simulink library "UXFD_Lib"  (R2016b)
settings: Solver=ode45  StartTime=0.0  StopTime=10.0  RelTol=1e-3  EnableMultiTasking=on
undefined symbols (not defined in the file): BreakpointData, BreakpointData1, BreakpointData2, BreakpointData_One_A, BreakpointData_Two_A, E2E_P01DataIDMode, E2E_P01ReceiverStatusType, EnumClass, iBit, initalValue, No_Runnable_Period, ObB_EidBsgStDerat_C, p_OVERRIDE_MASTER_SWITCH, SlDemoSign, SwitchOff_P, SwitchOn_P, Table, TableData_M, VCCTi33, VSysD_FidVehDerat1_C
libraries: simulink x28, CCMLib x11, UXFD_Lib x8, canmsglib x2, PTCC_Lib x1, hdlsllib x1
(part 5 of 7)

== system UXFD_Lib/Standard/Calibration/OverRide_with_master_switch ==
  override_value : Inport
  switch : Inport  Port=2
  input : Inport  Port=3
  Constant : Constant  Value=p_OVERRIDE_MASTER_SWITCH
  Constant1 : Constant  Value=85  OutDataTypeStr=uint8
  Data Type Conversion2 : DataTypeConversion  OutDataTypeStr=boolean
  Logical Operator : Logic
  Relational Operator1 : RelationalOperator  Operator===  OutDataTypeStr=boolean  RndMeth=Nearest  InputSameDT=on
  Switch1 : Switch  Criteria=u2 ~= 0  Threshold=1  RndMeth=Zero  InputSameDT=on
      settings: AttributesFormatString=%<Criteria>
  Out : Outport
  wires:
  Constant1/1 -> Relational Operator1/2
  Relational Operator1/1 -> Logical Operator/2
  input/1 -> Switch1/3
  Switch1/1 -> Out/1
  override_value/1 -> Switch1/1
  Data Type Conversion2/1 -> Switch1/2
  switch/1 -> Logical Operator/1
  Logical Operator/1 -> Data Type Conversion2/1
  Constant/1 -> Relational Operator1/1

== system UXFD_Lib/Standard/Calibration/xbackground1 ==

== system UXFD_Lib/Standard/Calibration/xbackground2 ==

== system UXFD_Lib/Standard/Calibration/xbackground3 ==

== system UXFD_Lib/Standard/Calibration/xbackground4 ==

== system UXFD_Lib/Standard/Discrete dynamics/BumplessRateTransfer ==
  s : Inport
  u1 : Inport  Port=2
  u0 : Inport  Port=3
  d10 : Inport  Port=4
  d01 : Inport  Port=5
  Add : Sum  Inputs=-+
  Add1 : Sum
  Constant1 : Constant  Value=0
  Constant2 : Constant
  LogicalSwitch1 : Subsystem  mask(GL_LogicSwitch_1.0){}
      mask init:
      | set_param(gcb,'LinkStatus','none');
      mask Display:
      | plot([-0.1 0.2 0.2], [0.85 0.85 0.75])
      | plot([-0.1 0.2 0.2], [0.5 0.5 0.6])
      | plot([0.8 1.1], [0.5 0.5])
      | plot([0.15 0.8], [0.6 0.5])
      | plot([-0.1 0.5 0.5], [0.15 0.15 0.6])
  Product : Product
  RateLimit : Subsystem  mask(PAG_Rate_Limiter_LV1.1_BV2){}
      mask help:
      | Rate limiter.
      | Limits the derivative of the input signal to a
      | value beween df (fall rate) and dr (rise rate).
      mask Display:
      | plot([0.35, 0.55, 0.55, 1.0], [0, 0, 1, 1])
      | plot([0.35, 0.55, 0.8, 1.0], [0, 0, 1, 1])
  Tq_EngInstReq_ : Outport
  wires:
  Add/1 -> Product/1
  Product/1 -> Add1/2
  Add1/1 -> Tq_EngInstReq_/1
  u0/1 -> Add1/1, Add/1
  u1/1 -> Add/2
  s/1 -> LogicalSwitch1/3(In3)
  Constant2/1 -> LogicalSwitch1/1(In1)
  Constant1/1 -> LogicalSwitch1/2(In2)
  d10/1 -> RateLimit/3(df)
  d01/1 -> RateLimit/2(dr)
  LogicalSwitch1/1(Out1) -> RateLimit/1(In1)
  RateLimit/1(y) -> Product/2

== system UXFD_Lib/Standard/Discrete dynamics/BumplessTransfer ==
  s : Inport
  u1 : Inport  Port=2
  u0 : Inport  Port=3
  tc : Inport  Port=4
  Add : Sum  Inputs=-+
  Add1 : Sum
  Constant : Constant  Value=0  OutDataTypeStr=Inherit: Inherit via back propagation
  Constant1 : Constant  OutDataTypeStr=Inherit: Inherit via back propagation
  LPF1_pole1 : Subsystem  mask(PAG_FirstOrder_Lowpass_Filter_LV1.1_BV2){}
      mask help:
      | Discrete low-pass filter. Corresponding analogue transfer function:
      |   1 / (1 + tau * s)
      mask Display:
      | plot([0.35, 0.9], [0, 0], [0.35, 0.35], [0, 1])
      | plot(0.35:0.55/10:0.9,   [0 0.39 0.63 0.78 0.86 0.92 0.95 0.98 0.99 0.99 0.99])
  LogicalSwitch1 : Subsystem  mask(GL_LogicSwitch_1.0){}
      mask init:
      | set_param(gcb,'LinkStatus','none');
      mask Display:
      | plot([-0.1 0.2 0.2], [0.85 0.85 0.75])
      | plot([-0.1 0.2 0.2], [0.5 0.5 0.6])
      | plot([0.8 1.1], [0.5 0.5])
      | plot([0.15 0.8], [0.6 0.5])
      | plot([-0.1 0.5 0.5], [0.15 0.15 0.6])
  Product : Product
  Out : Outport
  wires:
  Add/1 -> Product/1
  u0/1 -> Add1/1, Add/1
  s/1 -> LogicalSwitch1/3(In3)
  Product/1 -> Add1/2
  Add1/1 -> Out/1
  u1/1 -> Add/2
  LogicalSwitch1/1(Out1) -> LPF1_pole1/1(u)
  Constant1/1 -> LogicalSwitch1/1(In1)
  Constant/1 -> LogicalSwitch1/2(In2)
  LPF1_pole1/1(y) -> Product/2
  tc/1 -> LPF1_pole1/2(tc)

== system UXFD_Lib/Standard/Discrete dynamics/DLPF1_pole_v2 ==
  u : Inport
  tc : Inport  Port=2
  Add : Sum
  Add1 : Sum  Inputs=-+
  Add2 : Sum
  Add3 : Sum  Inputs=+-
  Constant : Constant  Value=0
  Constant1 : Constant  Value=0
  Constant2 : Constant  Value=1e-6
  Constant3 : Constant  Value=1e-6
  Divide : Product  Inputs=*/
  Divide1 : Product  Inputs=*/
  LogicalSwitch1 : Subsystem  mask(GL_LogicSwitch_1.0){}
      mask init:
      | set_param(gcb,'LinkStatus','none');
      mask Display:
      | plot([-0.1 0.2 0.2], [0.85 0.85 0.75])
      | plot([-0.1 0.2 0.2], [0.5 0.5 0.6])
      | plot([0.8 1.1], [0.5 0.5])
      | plot([0.15 0.8], [0.6 0.5])
      | plot([-0.1 0.5 0.5], [0.15 0.15 0.6])
  MinMax : MinMax  Function=max  Inputs=2
  MinMax1 : MinMax  Function=max  Inputs=2
  Product : Product
  Unit Delay : UnitDelay  SampleTime=-1
  Unit Delay1 : UnitDelay  SampleTime=-1
  Unit Delay2 : UnitDelay  SampleTime=-1
  ts : DataStoreRead  DataStoreName=ts
  y : Outport
  wires:
  tc/1 -> Add2/2
  MinMax1/1 -> Divide/2
  Constant3/1 -> MinMax1/2
  Add2/1 -> MinMax1/1
  u/1 -> Add3/1, Unit Delay/1
  Unit Delay/1 -> Add3/2
  Add3/1 -> Divide1/1
  Product/1 -> Add/2
  Divide1/1 -> Add1/2
  Unit Delay1/1 -> Add1/1, Add/1
  Divide/1 -> Product/2
  Add1/1 -> Product/1
  MinMax/1 -> Divide1/2
  Constant2/1 -> MinMax/2
  ts/1 -> Add2/1, MinMax/1, Divide/1
  Unit Delay2/1 -> LogicalSwitch1/3(In3)
  Constant1/1 -> Unit Delay2/1
  Constant/1 -> LogicalSwitch1/1(In1)
  Add/1 -> LogicalSwitch1/2(In2)
  LogicalSwitch1/1(Out1) -> Unit Delay1/1, y/1

== system UXFD_Lib/Standard/Discrete dynamics/FirstOrderFilter ==
  u : Inport
  tc : Inport  Port=2
  Constant1 : Constant  Value=1e-6  OutDataTypeStr=single  mask(TL_Constant){data={'output',{'type','Float32'},'date',735300.29228814819}}
      settings: CopyFcn=if exist('tl_reset_reviewflag','file')==2,tl_reset_reviewflag(gcbh);end  DeleteFcn=if exist('delete_tlblock','file')==2,delete_tlblock(gcbh);end  NameChangeFcn=if exist('rename_tlblock','file')==2,rename_tlblock(gcbh);end  OpenFcn=if exist('tl_open_blockdlg','file')==2,tl_open_blockdlg(gcbh);else,open_system(gcbh,'parameter');end
      mask Help: eval(['if exist(''tl_online_help'',''file'') == 2, tl_online_help(''Topic'',''TL_Constant''),else, web([''jar:file:///'',matlabroot,''/help/toolbox/simulink/help.jar!/slref/' lower(get_param(gcbh,'Blocktype')) '.html''], ''-helpbrowser''),end'])
      mask Display: plot([-0.05, 1.05, NaN, -0.05, 1.05],[.01, .01, NaN, .99, .99])
  Del1 : UnitDelay  SampleTime=-1  mask(TL_UnitDelay){data={'logdata',{'maxnumvals',4096,'plotchannels',[]},'output',{'type','Float32'},'state',{'type','Float32'},'date',735300.29228789348}}
      settings: CopyFcn=if exist('tl_reset_reviewflag','file')==2,tl_reset_reviewflag(gcbh);end  DeleteFcn=if exist('delete_tlblock','file')==2,delete_tlblock(gcbh);end  NameChangeFcn=if exist('rename_tlblock','file')==2,rename_tlblock(gcbh);end  OpenFcn=if exist('tl_open_blockdlg','file')==2,tl_open_blockdlg(gcbh);else,open_system(gcbh,'parameter');end
      mask Help: eval(['if exist(''tl_online_help'',''file'') == 2, tl_online_help(''Topic'',''TL_UnitDelay''),else, web([''jar:file:///'',matlabroot,''/help/toolbox/simulink/help.jar!/slref/' lower(get_param(gcbh,'Blocktype')) '.html''], ''-helpbrowser''),end'])
      mask Display: plot([-0.05, 1.05, NaN, -0.05, 1.05],[.01, .01, NaN, .99, .99])
  MinMax : MinMax  Function=max  Inputs=3  InputSameDT=on  mask(TL_MinMax){data={'logdata',{'maxnumvals',4096,'plotchannels',[]},'output',{'type','Float32'},'date',735300.29228754633}}
      settings: CopyFcn=if exist('tl_reset_reviewflag','file')==2,tl_reset_reviewflag(gcbh);end  DeleteFcn=if exist('delete_tlblock','file')==2,delete_tlblock(gcbh);end  NameChangeFcn=if exist('rename_tlblock','file')==2,rename_tlblock(gcbh);end  OpenFcn=if exist('tl_open_blockdlg','file')==2,tl_open_blockdlg(gcbh);else,open_system(gcbh,'parameter');end
      mask Help: eval(['if exist(''tl_online_help'',''file'') == 2, tl_online_help(''Topic'',''TL_MinMax''),else, web([''jar:file:///'',matlabroot,''/help/toolbox/simulink/help.jar!/slref/' lower(get_param(gcbh,'Blocktype')) '.html''], ''-helpbrowser''),end'])
      mask Display: plot([-0.05, 1.05, NaN, -0.05, 1.05],[.01, .01, NaN, .99, .99])
  Prod1 : Product  Inputs=*/  RndMeth=Zero  InputSameDT=on  OutDataTypeStr=Inherit: Same as first input  mask(TL_Product){data={'logdata',{'maxnumvals',4096,'plotchannels',[]},'output',{'type','Float32'},'date',735300.29228725692}}
      settings: CopyFcn=if exist('tl_reset_reviewflag','file')==2,tl_reset_reviewflag(gcbh);end  DeleteFcn=if exist('delete_tlblock','file')==2,delete_tlblock(gcbh);end  NameChangeFcn=if exist('rename_tlblock','file')==2,rename_tlblock(gcbh);end  OpenFcn=if exist('tl_open_blockdlg','file')==2,tl_open_blockdlg(gcbh);else,open_system(gcbh,'parameter');end
      mask Help: eval(['if exist(''tl_online_help'',''file'') == 2, tl_online_help(''Topic'',''TL_Product''),else, web([''jar:file:///'',matlabroot,''/help/toolbox/simulink/help.jar!/slref/' lower(get_param(gcbh,'Blocktype')) '.html''], ''-helpbrowser''),end'])
      mask Display: plot([-0.05, 1.05, NaN, -0.05, 1.05],[.01, .01, NaN, .99, .99])
  Prod2 : Product  RndMeth=Zero  InputSameDT=on  OutDataTypeStr=Inherit: Same as first input  mask(TL_Product){data={'logdata',{'maxnumvals',4096,'plotchannels',[]},'output',{'type','Float32'},'date',735300.29228697915}}
      settings: CopyFcn=if exist('tl_reset_reviewflag','file')==2,tl_reset_reviewflag(gcbh);end  DeleteFcn=if exist('delete_tlblock','file')==2,delete_tlblock(gcbh);end  NameChangeFcn=if exist('rename_tlblock','file')==2,rename_tlblock(gcbh);end  OpenFcn=if exist('tl_open_blockdlg','file')==2,tl_open_blockdlg(gcbh);else,open_system(gcbh,'parameter');end
      mask Help: eval(['if exist(''tl_online_help'',''file'') == 2, tl_online_help(''Topic'',''TL_Product''),else, web([''jar:file:///'',matlabroot,''/help/toolbox/simulink/help.jar!/slref/' lower(get_param(gcbh,'Blocktype')) '.html''], ''-helpbrowser''),end'])
      mask Display: plot([-0.05, 1.05, NaN, -0.05, 1.05],[.01, .01, NaN, .99, .99])
  Sum1 : Sum  Inputs=-+  InputSameDT=on  OutDataTypeStr=Inherit: Same as first input  mask(TL_Sum){data={'logdata',{'maxnumvals',4096,'plotchannels',[]},'output',{'type','Float32'},'date',735300.29228671291}}
      settings: CopyFcn=if exist('tl_reset_reviewflag','file')==2,tl_reset_reviewflag(gcbh);end  DeleteFcn=if exist('delete_tlblock','file')==2,delete_tlblock(gcbh);end  NameChangeFcn=if exist('rename_tlblock','file')==2,rename_tlblock(gcbh);end  OpenFcn=if exist('tl_open_blockdlg','file')==2,tl_open_blockdlg(gcbh);else,open_system(gcbh,'parameter');end
      mask Help: eval(['if exist(''tl_online_help'',''file'') == 2, tl_online_help(''Topic'',''TL_Sum''),else, web([''jar:file:///'',matlabroot,''/help/toolbox/simulink/help.jar!/slref/' lower(get_param(gcbh,'Blocktype')) '.html''], ''-helpbrowser''),end'])
      mask Display: plot([-0.05, 1.05, NaN, -0.05, 1.05],[.01, .01, NaN, .99, .99])
  Sum2 : Sum  InputSameDT=on  OutDataTypeStr=Inherit: Same as first input  mask(TL_Sum){data={'logdata',{'maxnumvals',4096,'plotchannels',[]},'output',{'type','Float32'},'date',735300.29228643514}}
      settings: CopyFcn=if exist('tl_reset_reviewflag','file')==2,tl_reset_reviewflag(gcbh);end  DeleteFcn=if exist('delete_tlblock','file')==2,delete_tlblock(gcbh);end  NameChangeFcn=if exist('rename_tlblock','file')==2,rename_tlblock(gcbh);end  OpenFcn=if exist('tl_open_blockdlg','file')==2,tl_open_blockdlg(gcbh);else,open_system(gcbh,'parameter');end
      mask Help: eval(['if exist(''tl_online_help'',''file'') == 2, tl_online_help(''Topic'',''TL_Sum''),else, web([''jar:file:///'',matlabroot,''/help/toolbox/simulink/help.jar!/slref/' lower(get_param(gcbh,'Blocktype')) '.html''], ''-helpbrowser''),end'])
      mask Display: plot([-0.05, 1.05, NaN, -0.05, 1.05],[.01, .01, NaN, .99, .99])
  ts : UXFD_Lib/Standard/Discrete dynamics/FirstOrderFilter1/ts  data={'logdata',{'plotchannels',[]},'date',735300.29228288191}
      settings: AttributesFormatString=ts
  y : Outport
  wires:
  u/1 -> Sum1/2
  Sum1/1 -> Prod2/1
  MinMax/1 -> Prod1/2
  ts/1 -> Prod1/1, MinMax/1
  Prod1/1 -> Prod2/2
  Del1/1 -> Sum1/1, Sum2/1
  Sum2/1 -> y/1, Del1/1
  tc/1 -> MinMax/2
  Prod2/1 -> Sum2/2
  Constant1/1 -> MinMax/3

== system UXFD_Lib/Standard/Discrete dynamics/FirstOrderFilter1 ==
  u : Inport
  r : Inport  Port=2
  rv : Inport  Port=3
  tc inc : Inport  Port=4
  tc dec : Inport  Port=5
  Constant : Constant  Value=0  mask(TL_Constant){data={'output',{'type','Float32'},'date',735300.29228606483}}
      settings: CopyFcn=if exist('tl_reset_reviewflag','file')==2,tl_reset_reviewflag(gcbh);end  DeleteFcn=if exist('delete_tlblock','file')==2,delete_tlblock(gcbh);end  NameChangeFcn=if exist('rename_tlblock','file')==2,rename_tlblock(gcbh);end  OpenFcn=if exist('tl_open_blockdlg','file')==2,tl_open_blockdlg(gcbh);else,open_system(gcbh,'parameter');end
      mask Help: eval(['if exist(''tl_online_help'',''file'') == 2, tl_online_help(''Topic'',''TL_Constant''),else, web([''jar:file:///'',matlabroot,''/help/toolbox/simulink/help.jar!/slref/' lower(get_param(gcbh,'Blocktype')) '.html''], ''-helpbrowser''),end'])
      mask Display: plot([-0.05, 1.05, NaN, -0.05, 1.05],[.01, .01, NaN, .99, .99])
  Constant1 : Constant  Value=1e-6  OutDataTypeStr=single  mask(TL_Constant){data={'output',{'type','Float32'},'date',735300.29228582175}}
      settings: CopyFcn=if exist('tl_reset_reviewflag','file')==2,tl_reset_reviewflag(gcbh);end  DeleteFcn=if exist('delete_tlblock','file')==2,delete_tlblock(gcbh);end  NameChangeFcn=if exist('rename_tlblock','file')==2,rename_tlblock(gcbh);end  OpenFcn=if exist('tl_open_blockdlg','file')==2,tl_open_blockdlg(gcbh);else,open_system(gcbh,'parameter');end
      mask Help: eval(['if exist(''tl_online_help'',''file'') == 2, tl_online_help(''Topic'',''TL_Constant''),else, web([''jar:file:///'',matlabroot,''/help/toolbox/simulink/help.jar!/slref/' lower(get_param(gcbh,'Blocktype')) '.html''], ''-helpbrowser''),end'])
      mask Display: plot([-0.05, 1.05, NaN, -0.05, 1.05],[.01, .01, NaN, .99, .99])
  Del1 : UnitDelay  SampleTime=-1  mask(TL_UnitDelay){data={'logdata',{'maxnumvals',4096,'plotchannels',[]},'output',{'type','Float32'},'state',{'type','Float32'},'date',735300.29228555551}}
      settings: CopyFcn=if exist('tl_reset_reviewflag','file')==2,tl_reset_reviewflag(gcbh);end  DeleteFcn=if exist('delete_tlblock','file')==2,delete_tlblock(gcbh);end  NameChangeFcn=if exist('rename_tlblock','file')==2,rename_tlblock(gcbh);end  OpenFcn=if exist('tl_open_blockdlg','file')==2,tl_open_blockdlg(gcbh);else,open_system(gcbh,'parameter');end
      mask Help: eval(['if exist(''tl_online_help'',''file'') == 2, tl_online_help(''Topic'',''TL_UnitDelay''),else, web([''jar:file:///'',matlabroot,''/help/toolbox/simulink/help.jar!/slref/' lower(get_param(gcbh,'Blocktype')) '.html''], ''-helpbrowser''),end'])
      mask Display: plot([-0.05, 1.05, NaN, -0.05, 1.05],[.01, .01, NaN, .99, .99])
  Demux : Demux  Outputs=2
  Max2 : MinMax  Function=max  Inputs=2  mask(TL_MinMax){data={'logdata',{'plotchannels',[]},'output',{'type','Float32'},'date',735300.29228521988}}
      settings: CopyFcn=if exist('tl_reset_reviewflag','file')==2,tl_reset_reviewflag(gcbh);end  DeleteFcn=if exist('delete_tlblock','file')==2,delete_tlblock(gcbh);end  NameChangeFcn=if exist('rename_tlblock','file')==2,rename_tlblock(gcbh);end  OpenFcn=if exist('tl_open_blockdlg','file')==2,tl_open_blockdlg(gcbh);else,open_system(gcbh,'parameter');end
      mask Help: eval(['if exist(''tl_online_help'',''file'') == 2, tl_online_help(''Topic'',''TL_MinMax''),else, web([''jar:file:///'',matlabroot,''/help/toolbox/simulink/help.jar!/slref/' lower(get_param(gcbh,'Blocktype')) '.html''], ''-helpbrowser''),end'])
      mask Display: plot([-0.05, 1.05, NaN, -0.05, 1.05],[.01, .01, NaN, .99, .99])
  Min : MinMax  Inputs=2  mask(TL_MinMax){data={'logdata',{'plotchannels',[]},'output',{'type','Float32'},'date',735300.29228494212}}
      settings: CopyFcn=if exist('tl_reset_reviewflag','file')==2,tl_reset_reviewflag(gcbh);end  DeleteFcn=if exist('delete_tlblock','file')==2,delete_tlblock(gcbh);end  NameChangeFcn=if exist('rename_tlblock','file')==2,rename_tlblock(gcbh);end  OpenFcn=if exist('tl_open_blockdlg','file')==2,tl_open_blockdlg(gcbh);else,open_system(gcbh,'parameter');end
      mask Help: eval(['if exist(''tl_online_help'',''file'') == 2, tl_online_help(''Topic'',''TL_MinMax''),else, web([''jar:file:///'',matlabroot,''/help/toolbox/simulink/help.jar!/slref/' lower(get_param(gcbh,'Blocktype')) '.html''], ''-helpbrowser''),end'])
      mask Display: plot([-0.05, 1.05, NaN, -0.05, 1.05],[.01, .01, NaN, .99, .99])
  MinMax : MinMax  Function=max  Inputs=3  InputSameDT=on  mask(TL_MinMax){data={'logdata',{'maxnumvals',4096,'plotchannels',[]},'output',{'type','Float32'},'date',735300.29228465282}}
      settings: CopyFcn=if exist('tl_reset_reviewflag','file')==2,tl_reset_reviewflag(gcbh);end  DeleteFcn=if exist('delete_tlblock','file')==2,delete_tlblock(gcbh);end  NameChangeFcn=if exist('rename_tlblock','file')==2,rename_tlblock(gcbh);end  OpenFcn=if exist('tl_open_blockdlg','file')==2,tl_open_blockdlg(gcbh);else,open_system(gcbh,'parameter');end
      mask Help: eval(['if exist(''tl_online_help'',''file'') == 2, tl_online_help(''Topic'',''TL_MinMax''),else, web([''jar:file:///'',matlabroot,''/help/toolbox/simulink/help.jar!/slref/' lower(get_param(gcbh,'Blocktype')) '.html''], ''-helpbrowser''),end'])
      mask Display: plot([-0.05, 1.05, NaN, -0.05, 1.05],[.01, .01, NaN, .99, .99])
  Mux : Mux  Inputs=2
  Mux1 : Mux  Inputs=2
  Prod1 : Product  Inputs=*/  RndMeth=Zero  InputSameDT=on  OutDataTypeStr=Inherit: Same as first input  mask(TL_Product){data={'logdata',{'maxnumvals',4096,'plotchannels',[]},'output',{'type','Float32'},'date',735300.29228437506}}
      settings: CopyFcn=if exist('tl_reset_reviewflag','file')==2,tl_reset_reviewflag(gcbh);end  DeleteFcn=if exist('delete_tlblock','file')==2,delete_tlblock(gcbh);end  NameChangeFcn=if exist('rename_tlblock','file')==2,rename_tlblock(gcbh);end  OpenFcn=if exist('tl_open_blockdlg','file')==2,tl_open_blockdlg(gcbh);else,open_system(gcbh,'parameter');end
      mask Help: eval(['if exist(''tl_online_help'',''file'') == 2, tl_online_help(''Topic'',''TL_Product''),else, web([''jar:file:///'',matlabroot,''/help/toolbox/simulink/help.jar!/slref/' lower(get_param(gcbh,'Blocktype')) '.html''], ''-helpbrowser''),end'])
      mask Display: plot([-0.05, 1.05, NaN, -0.05, 1.05],[.01, .01, NaN, .99, .99])
  Prod2 : Product  RndMeth=Zero  InputSameDT=on  OutDataTypeStr=Inherit: Same as first input  mask(TL_Product){data={'logdata',{'maxnumvals',4096,'plotchannels',[]},'output',{'type','Float32'},'date',735300.29228409717}}
      settings: CopyFcn=if exist('tl_reset_reviewflag','file')==2,tl_reset_reviewflag(gcbh);end  DeleteFcn=if exist('delete_tlblock','file')==2,delete_tlblock(gcbh);end  NameChangeFcn=if exist('rename_tlblock','file')==2,rename_tlblock(gcbh);end  OpenFcn=if exist('tl_open_blockdlg','file')==2,tl_open_blockdlg(gcbh);else,open_system(gcbh,'parameter');end
      mask Help: eval(['if exist(''tl_online_help'',''file'') == 2, tl_online_help(''Topic'',''TL_Product''),else, web([''jar:file:///'',matlabroot,''/help/toolbox/simulink/help.jar!/slref/' lower(get_param(gcbh,'Blocktype')) '.html''], ''-helpbrowser''),end'])
      mask Display: plot([-0.05, 1.05, NaN, -0.05, 1.05],[.01, .01, NaN, .99, .99])
  Sum1 : Sum  Inputs=-+  InputSameDT=on  OutDataTypeStr=Inherit: Same as first input  mask(TL_Sum){data={'logdata',{'maxnumvals',4096,'plotchannels',[]},'output',{'type','Float32'},'date',735300.29228373838}}
      settings: CopyFcn=if exist('tl_reset_reviewflag','file')==2,tl_reset_reviewflag(gcbh);end  DeleteFcn=if exist('delete_tlblock','file')==2,delete_tlblock(gcbh);end  NameChangeFcn=if exist('rename_tlblock','file')==2,rename_tlblock(gcbh);end  OpenFcn=if exist('tl_open_blockdlg','file')==2,tl_open_blockdlg(gcbh);else,open_system(gcbh,'parameter');end
      mask Help: eval(['if exist(''tl_online_help'',''file'') == 2, tl_online_help(''Topic'',''TL_Sum''),else, web([''jar:file:///'',matlabroot,''/help/toolbox/simulink/help.jar!/slref/' lower(get_param(gcbh,'Blocktype')) '.html''], ''-helpbrowser''),end'])
      mask Display: plot([-0.05, 1.05, NaN, -0.05, 1.05],[.01, .01, NaN, .99, .99])
  Sum2 : Sum  Inputs=+++  InputSameDT=on  OutDataTypeStr=Inherit: Same as first input  mask(TL_Sum){data={'logdata',{'maxnumvals',4096,'plotchannels',[]},'output',{'type','Float32'},'date',735300.29228347226}}
      settings: CopyFcn=if exist('tl_reset_reviewflag','file')==2,tl_reset_reviewflag(gcbh);end  DeleteFcn=if exist('delete_tlblock','file')==2,delete_tlblock(gcbh);end  NameChangeFcn=if exist('rename_tlblock','file')==2,rename_tlblock(gcbh);end  OpenFcn=if exist('tl_open_blockdlg','file')==2,tl_open_blockdlg(gcbh);else,open_system(gcbh,'parameter');end
      mask Help: eval(['if exist(''tl_online_help'',''file'') == 2, tl_online_help(''Topic'',''TL_Sum''),else, web([''jar:file:///'',matlabroot,''/help/toolbox/simulink/help.jar!/slref/' lower(get_param(gcbh,'Blocktype')) '.html''], ''-helpbrowser''),end'])
      mask Display: plot([-0.05, 1.05, NaN, -0.05, 1.05],[.01, .01, NaN, .99, .99])
  Switch : Switch  Criteria=u2 ~= 0  Threshold=0.5  mask(TL_Switch){data={'logdata',{'plotchannels',[]},'output',{'type','Float32'},'date',735300.29228318285}}
      settings: CopyFcn=if exist('tl_reset_reviewflag','file')==2,tl_reset_reviewflag(gcbh);end  DeleteFcn=if exist('delete_tlblock','file')==2,delete_tlblock(gcbh);end  NameChangeFcn=if exist('rename_tlblock','file')==2,rename_tlblock(gcbh);end  OpenFcn=if exist('tl_open_blockdlg','file')==2,tl_open_blockdlg(gcbh);else,open_system(gcbh,'parameter');end
      mask Help: eval(['if exist(''tl_online_help'',''file'') == 2, tl_online_help(''Topic'',''TL_Switch''),else, web([''jar:file:///'',matlabroot,''/help/toolbox/simulink/help.jar!/slref/' lower(get_param(gcbh,'Blocktype')) '.html''], ''-helpbrowser''),end'])
      mask Display: plot([-0.05, 1.05, NaN, -0.05, 1.05],[.01, .01, NaN, .99, .99])
  ts : DataStoreRead  DataStoreName=ts  mask(TL_DataStoreRead){data={'logdata',{'plotchannels',[]},'date',735300.29228288191}}
      settings: AttributesFormatString=ts  DeleteFcn=if exist('delete_tlblock','file')==2,delete_tlblock(gcbh);end  NameChangeFcn=if exist('rename_tlblock','file')==2,rename_tlblock(gcbh);end  OpenFcn=if exist('tl_open_blockdlg','file')==2,tl_open_blockdlg(gcbh);else,open_system(gcbh,'parameter');end
      mask Help: eval(['if exist(''tl_online_help'',''file'') == 2, tl_online_help(''Topic'',''TL_DataStoreRead''),else, web([''jar:file:///'',matlabroot,''/help/toolbox/simulink/help.jar!/slref/' lower(get_param(gcbh,'Blocktype')) '.html''], ''-helpbrowser''),end'])
      mask Display: plot([-0.05, 1.05, NaN, -0.05, 1.05],[.01, .01, NaN, .99, .99])
  y : Outport
  wires:
  Del1/1 -> Sum2/1, Sum1/1
  Prod1/1 -> Prod2/2
  ts/1 -> Prod1/1, MinMax/1
  MinMax/1 -> Prod1/2
  Sum1/1 -> Prod2/1
  u/1 -> Sum1/2
  tc inc/1 -> Mux/1
  tc dec/1 -> Mux/2
  Constant1/1 -> Mux1/1, Mux1/2
  Prod2/1 -> Demux/1
  Demux/1 -> Max2/1
  Demux/2 -> Min/2
  Constant/1 -> Max2/2, Min/1
  Max2/1 -> Sum2/2
  Min/1 -> Sum2/3
  Sum2/1 -> Switch/3
  rv/1 -> Switch/1
  r/1 -> Switch/2
  Switch/1 -> Del1/1, y/1
  Mux/1 -> MinMax/2
  Mux1/1 -> MinMax/3

== system UXFD_Lib/Standard/Discrete dynamics/HysteresisFilter ==
  note: Filter to avoid occilation during low slipp
      | when converter character is steep
  n_Eng5 : Inport
  n_Eng1 : Inport  Port=2
  Add : Sum
  Add1 : Sum  Inputs=+-
  Saturation1 : Subsystem  mask(GL_Saturation_1.0){}
      mask help:
      | If input_1 > input_2
      |   output = input_2
      | elseif input_1 < input_3
      |   output = input_3
      | else
      |   output = input_1
      |
      | Note that if the lower limit is set above the upper limit, the output will take the value of the input to the lower limit port.
      mask init:
      | set_param(gcb,'LinkStatus','none');
      mask Display: plot([0.3, 0.5, 0.7, 0.9], [0, 0, 1, 1])
  Unit Delay : UnitDelay  SampleTime=-1
  y : Outport
  wires:
  n_Eng5/1 -> Add/1, Add1/1
  Add1/1 -> Saturation1/3(L)
  Add/1 -> Saturation1/2(U)
  Saturation1/1(y) -> Unit Delay/1, y/1
  Unit Delay/1 -> Saturation1/1(u)
  n_Eng1/1 -> Add/2, Add1/2

== system UXFD_Lib/Standard/Discrete dynamics/LPF1_discreteReset ==
  u : Inport
  a : Inport  Port=2
  r : Inport  Port=3
  LogicalSwitch1 : Subsystem  mask(PAG_Switch_LV1.6_BV2){}
      mask help:
      | Pass through input 1 when input 3 is true;
      | otherwise, pass through input 2
      mask Display:
      | plot([-0.1 0.2 0.2], [0.85 0.85 0.75])
      | plot([-0.1 0.2 0.2], [0.5 0.5 0.6])
      | plot([0.8 1.1], [0.5 0.5])
      | plot([0.15 0.8], [0.6 0.5])
      | plot([-0.1 0.5 0.5], [0.15 0.15 0.6])
  Product : Product  SaturateOnIntegerOverflow=on  RndMeth=Zero  InputSameDT=on  OutDataTypeStr=Inherit: Same as first input  mask(TL_Product){data={'logdata',{'maxnumvals',4096,'plotchannels',[]},'output',{'type','Float32'},'date',735300.29228090274}}
      settings: CopyFcn=if exist('tl_reset_reviewflag','file')==2,tl_reset_reviewflag(gcbh);end  DeleteFcn=if exist('delete_tlblock','file')==2,delete_tlblock(gcbh);end  NameChangeFcn=if exist('rename_tlblock','file')==2,rename_tlblock(gcbh);end  OpenFcn=if exist('tl_open_blockdlg','file')==2,tl_open_blockdlg(gcbh);else,open_system(gcbh,'parameter');end
      mask Help: eval(['if exist(''tl_online_help'',''file'') == 2, tl_online_help(''Topic'',''TL_Product''),else, web([''jar:file:///'',matlabroot,''/help/toolbox/simulink/help.jar!/slref/' lower(get_param(gcbh,'Blocktype')) '.html''], ''-helpbrowser''),end'])
      mask Display: plot([-0.05, 1.05, NaN, -0.05, 1.05],[.01, .01, NaN, .99, .99])
  Sum : Sum  Inputs=+-  SaturateOnIntegerOverflow=on  InputSameDT=on  OutDataTypeStr=Inherit: Same as first input  mask(TL_Sum){data={'logdata',{'maxnumvals',4096,'plotchannels',[]},'output',{'type','Float32'},'date',735300.29228062497}}
      settings: CopyFcn=if exist('tl_reset_reviewflag','file')==2,tl_reset_reviewflag(gcbh);end  DeleteFcn=if exist('delete_tlblock','file')==2,delete_tlblock(gcbh);end  NameChangeFcn=if exist('rename_tlblock','file')==2,rename_tlblock(gcbh);end  OpenFcn=if exist('tl_open_blockdlg','file')==2,tl_open_blockdlg(gcbh);else,open_system(gcbh,'parameter');end
      mask Help: eval(['if exist(''tl_online_help'',''file'') == 2, tl_online_help(''Topic'',''TL_Sum''),else, web([''jar:file:///'',matlabroot,''/help/toolbox/simulink/help.jar!/slref/' lower(get_param(gcbh,'Blocktype')) '.html''], ''-helpbrowser''),end'])
      mask Display: plot([-0.05, 1.05, NaN, -0.05, 1.05],[.01, .01, NaN, .99, .99])
  Sum1 : Sum  SaturateOnIntegerOverflow=on  InputSameDT=on  OutDataTypeStr=Inherit: Same as first input  mask(TL_Sum){data={'logdata',{'maxnumvals',4096,'plotchannels',[]},'output',{'type','Float32'},'date',735300.2922803472}}
      settings: CopyFcn=if exist('tl_reset_reviewflag','file')==2,tl_reset_reviewflag(gcbh);end  DeleteFcn=if exist('delete_tlblock','file')==2,delete_tlblock(gcbh);end  NameChangeFcn=if exist('rename_tlblock','file')==2,rename_tlblock(gcbh);end  OpenFcn=if exist('tl_open_blockdlg','file')==2,tl_open_blockdlg(gcbh);else,open_system(gcbh,'parameter');end
      mask Help: eval(['if exist(''tl_online_help'',''file'') == 2, tl_online_help(''Topic'',''TL_Sum''),else, web([''jar:file:///'',matlabroot,''/help/toolbox/simulink/help.jar!/slref/' lower(get_param(gcbh,'Blocktype')) '.html''], ''-helpbrowser''),end'])
      mask Display: plot([-0.05, 1.05, NaN, -0.05, 1.05],[.01, .01, NaN, .99, .99])
  UnitDelay : UnitDelay  SampleTime=-1  mask(TL_UnitDelay){data={'logdata',{'maxnumvals',4096,'plotchannels',[]},'output',{'type','Float32'},'state',{'type','Float32'},'date',735300.29228006944}}
      settings: CopyFcn=if exist('tl_reset_reviewflag','file')==2,tl_reset_reviewflag(gcbh);end  DeleteFcn=if exist('delete_tlblock','file')==2,delete_tlblock(gcbh);end  NameChangeFcn=if exist('rename_tlblock','file')==2,rename_tlblock(gcbh);end  OpenFcn=if exist('tl_open_blockdlg','file')==2,tl_open_blockdlg(gcbh);else,open_system(gcbh,'parameter');end
      mask Help: eval(['if exist(''tl_online_help'',''file'') == 2, tl_online_help(''Topic'',''TL_UnitDelay''),else, web([''jar:file:///'',matlabroot,''/help/toolbox/simulink/help.jar!/slref/' lower(get_param(gcbh,'Blocktype')) '.html''], ''-helpbrowser''),end'])
      mask Display: plot([-0.05, 1.05, NaN, -0.05, 1.05],[.01, .01, NaN, .99, .99])
  y : Outport
  wires:
  Product/1 -> Sum1/1
  a/1 -> Product/2
  Sum/1 -> Product/1
  u/1 -> Sum/2, Sum1/2, LogicalSwitch1/1(In1)
  r/1 -> LogicalSwitch1/3(In2)
  UnitDelay/1 -> Sum/1
  Sum1/1 -> LogicalSwitch1/2(In3)
  LogicalSwitch1/1(Out1) -> y/1, UnitDelay/1

== system UXFD_Lib/Standard/Discrete dynamics/LPF2_discrete ==
  u : Inport
  a1 : Inport  Port=2
  a2 : Inport  Port=3
  b0 : Inport  Port=4
  b1 : Inport  Port=5
  b2 : Inport  Port=6
  Product : Product  SaturateOnIntegerOverflow=on  RndMeth=Zero  InputSameDT=on  OutDataTypeStr=Inherit: Same as first input  mask(TL_Product){data={'logdata',{'maxnumvals',4096,'plotchannels',[]},'output',{'type','Float32'},'date',735300.29227971064}}
      settings: CopyFcn=if exist('tl_reset_reviewflag','file')==2,tl_reset_reviewflag(gcbh);end  DeleteFcn=if exist('delete_tlblock','file')==2,delete_tlblock(gcbh);end  NameChangeFcn=if exist('rename_tlblock','file')==2,rename_tlblock(gcbh);end  OpenFcn=if exist('tl_open_blockdlg','file')==2,tl_open_blockdlg(gcbh);else,open_system(gcbh,'parameter');end
      mask Help: eval(['if exist(''tl_online_help'',''file'') == 2, tl_online_help(''Topic'',''TL_Product''),else, web([''jar:file:///'',matlabroot,''/help/toolbox/simulink/help.jar!/slref/' lower(get_param(gcbh,'Blocktype')) '.html''], ''-helpbrowser''),end'])
      mask Display: plot([-0.05, 1.05, NaN, -0.05, 1.05],[.01, .01, NaN, .99, .99])
  Product1 : Product  SaturateOnIntegerOverflow=on  RndMeth=Zero  InputSameDT=on  OutDataTypeStr=Inherit: Same as first input  mask(TL_Product){data={'logdata',{'maxnumvals',4096,'plotchannels',[]},'output',{'type','Float32'},'date',735300.29227943288}}
      settings: CopyFcn=if exist('tl_reset_reviewflag','file')==2,tl_reset_reviewflag(gcbh);end  DeleteFcn=if exist('delete_tlblock','file')==2,delete_tlblock(gcbh);end  NameChangeFcn=if exist('rename_tlblock','file')==2,rename_tlblock(gcbh);end  OpenFcn=if exist('tl_open_blockdlg','file')==2,tl_open_blockdlg(gcbh);else,open_system(gcbh,'parameter');end
      mask Help: eval(['if exist(''tl_online_help'',''file'') == 2, tl_online_help(''Topic'',''TL_Product''),else, web([''jar:file:///'',matlabroot,''/help/toolbox/simulink/help.jar!/slref/' lower(get_param(gcbh,'Blocktype')) '.html''], ''-helpbrowser''),end'])
      mask Display: plot([-0.05, 1.05, NaN, -0.05, 1.05],[.01, .01, NaN, .99, .99])
  Product2 : Product  SaturateOnIntegerOverflow=on  RndMeth=Zero  InputSameDT=on  OutDataTypeStr=Inherit: Same as first input  mask(TL_Product){data={'logdata',{'maxnumvals',4096,'plotchannels',[]},'output',{'type','Float32'},'date',735300.29227915511}}
      settings: CopyFcn=if exist('tl_reset_reviewflag','file')==2,tl_reset_reviewflag(gcbh);end  DeleteFcn=if exist('delete_tlblock','file')==2,delete_tlblock(gcbh);end  NameChangeFcn=if exist('rename_tlblock','file')==2,rename_tlblock(gcbh);end  OpenFcn=if exist('tl_open_blockdlg','file')==2,tl_open_blockdlg(gcbh);else,open_system(gcbh,'parameter');end
      mask Help: eval(['if exist(''tl_online_help'',''file'') == 2, tl_online_help(''Topic'',''TL_Product''),else, web([''jar:file:///'',matlabroot,''/help/toolbox/simulink/help.jar!/slref/' lower(get_param(gcbh,'Blocktype')) '.html''], ''-helpbrowser''),end'])
      mask Display: plot([-0.05, 1.05, NaN, -0.05, 1.05],[.01, .01, NaN, .99, .99])
  Product3 : Product  SaturateOnIntegerOverflow=on  RndMeth=Zero  InputSameDT=on  OutDataTypeStr=Inherit: Same as first input  mask(TL_Product){data={'logdata',{'maxnumvals',4096,'plotchannels',[]},'output',{'type','Float32'},'date',735300.29227888887}}
      settings: CopyFcn=if exist('tl_reset_reviewflag','file')==2,tl_reset_reviewflag(gcbh);end  DeleteFcn=if exist('delete_tlblock','file')==2,delete_tlblock(gcbh);end  NameChangeFcn=if exist('rename_tlblock','file')==2,rename_tlblock(gcbh);end  OpenFcn=if exist('tl_open_blockdlg','file')==2,tl_open_blockdlg(gcbh);else,open_system(gcbh,'parameter');end
      mask Help: eval(['if exist(''tl_online_help'',''file'') == 2, tl_online_help(''Topic'',''TL_Product''),else, web([''jar:file:///'',matlabroot,''/help/toolbox/simulink/help.jar!/slref/' lower(get_param(gcbh,'Blocktype')) '.html''], ''-helpbrowser''),end'])
      mask Display: plot([-0.05, 1.05, NaN, -0.05, 1.05],[.01, .01, NaN, .99, .99])
  Product4 : Product  SaturateOnIntegerOverflow=on  RndMeth=Zero  InputSameDT=on  OutDataTypeStr=Inherit: Same as first input  mask(TL_Product){data={'logdata',{'maxnumvals',4096,'plotchannels',[]},'output',{'type','Float32'},'date',735300.2922786111}}
      settings: CopyFcn=if exist('tl_reset_reviewflag','file')==2,tl_reset_reviewflag(gcbh);end  DeleteFcn=if exist('delete_tlblock','file')==2,delete_tlblock(gcbh);end  NameChangeFcn=if exist('rename_tlblock','file')==2,rename_tlblock(gcbh);end  OpenFcn=if exist('tl_open_blockdlg','file')==2,tl_open_blockdlg(gcbh);else,open_system(gcbh,'parameter');end
      mask Help: eval(['if exist(''tl_online_help'',''file'') == 2, tl_online_help(''Topic'',''TL_Product''),else, web([''jar:file:///'',matlabroot,''/help/toolbox/simulink/help.jar!/slref/' lower(get_param(gcbh,'Blocktype')) '.html''], ''-helpbrowser''),end'])
      mask Display: plot([-0.05, 1.05, NaN, -0.05, 1.05],[.01, .01, NaN, .99, .99])
  Sum : Sum  Inputs=+++--  SaturateOnIntegerOverflow=on  InputSameDT=on  OutDataTypeStr=Inherit: Same as first input  mask(TL_Sum){data={'logdata',{'maxnumvals',4096,'plotchannels',[]},'output',{'type','Float32'},'date',735300.29227833333}}
      settings: CopyFcn=if exist('tl_reset_reviewflag','file')==2,tl_reset_reviewflag(gcbh);end  DeleteFcn=if exist('delete_tlblock','file')==2,delete_tlblock(gcbh);end  NameChangeFcn=if exist('rename_tlblock','file')==2,rename_tlblock(gcbh);end  OpenFcn=if exist('tl_open_blockdlg','file')==2,tl_open_blockdlg(gcbh);else,open_system(gcbh,'parameter');end
      mask Help: eval(['if exist(''tl_online_help'',''file'') == 2, tl_online_help(''Topic'',''TL_Sum''),else, web([''jar:file:///'',matlabroot,''/help/toolbox/simulink/help.jar!/slref/' lower(get_param(gcbh,'Blocktype')) '.html''], ''-helpbrowser''),end'])
      mask Display: plot([-0.05, 1.05, NaN, -0.05, 1.05],[.01, .01, NaN, .99, .99])
  UnitDelay : UnitDelay  SampleTime=-1  mask(TL_UnitDelay){data={'logdata',{'maxnumvals',4096,'plotchannels',[]},'output',{'type','Float32'},'state',{'type','Float32'},'date',735300.29227804393}}
      settings: CopyFcn=if exist('tl_reset_reviewflag','file')==2,tl_reset_reviewflag(gcbh);end  DeleteFcn=if exist('delete_tlblock','file')==2,delete_tlblock(gcbh);end  NameChangeFcn=if exist('rename_tlblock','file')==2,rename_tlblock(gcbh);end  OpenFcn=if exist('tl_open_blockdlg','file')==2,tl_open_blockdlg(gcbh);else,open_system(gcbh,'parameter');end
      mask Help: eval(['if exist(''tl_online_help'',''file'') == 2, tl_online_help(''Topic'',''TL_UnitDelay''),else, web([''jar:file:///'',matlabroot,''/help/toolbox/simulink/help.jar!/slref/' lower(get_param(gcbh,'Blocktype')) '.html''], ''-helpbrowser''),end'])
      mask Display: plot([-0.05, 1.05, NaN, -0.05, 1.05],[.01, .01, NaN, .99, .99])
  UnitDelay1 : UnitDelay  SampleTime=-1  mask(TL_UnitDelay){data={'logdata',{'maxnumvals',4096,'plotchannels',[]},'output',{'type','Float32'},'state',{'type','Float32'},'date',735300.29227769678}}
      settings: CopyFcn=if exist('tl_reset_reviewflag','file')==2,tl_reset_reviewflag(gcbh);end  DeleteFcn=if exist('delete_tlblock','file')==2,delete_tlblock(gcbh);end  NameChangeFcn=if exist('rename_tlblock','file')==2,rename_tlblock(gcbh);end  OpenFcn=if exist('tl_open_blockdlg','file')==2,tl_open_blockdlg(gcbh);else,open_system(gcbh,'parameter');end
      mask Help: eval(['if exist(''tl_online_help'',''file'') == 2, tl_online_help(''Topic'',''TL_UnitDelay''),else, web([''jar:file:///'',matlabroot,''/help/toolbox/simulink/help.jar!/slref/' lower(get_param(gcbh,'Blocktype')) '.html''], ''-helpbrowser''),end'])
      mask Display: plot([-0.05, 1.05, NaN, -0.05, 1.05],[.01, .01, NaN, .99, .99])
  UnitDelay2 : UnitDelay  SampleTime=-1  mask(TL_UnitDelay){data={'logdata',{'maxnumvals',4096,'plotchannels',[]},'output',{'type','Float32'},'state',{'type','Float32'},'date',735300.29227733798}}
      settings: CopyFcn=if exist('tl_reset_reviewflag','file')==2,tl_reset_reviewflag(gcbh);end  DeleteFcn=if exist('delete_tlblock','file')==2,delete_tlblock(gcbh);end  NameChangeFcn=if exist('rename_tlblock','file')==2,rename_tlblock(gcbh);end  OpenFcn=if exist('tl_open_blockdlg','file')==2,tl_open_blockdlg(gcbh);else,open_system(gcbh,'parameter');end
      mask Help: eval(['if exist(''tl_online_help'',''file'') == 2, tl_online_help(''Topic'',''TL_UnitDelay''),else, web([''jar:file:///'',matlabroot,''/help/toolbox/simulink/help.jar!/slref/' lower(get_param(gcbh,'Blocktype')) '.html''], ''-helpbrowser''),end'])
      mask Display: plot([-0.05, 1.05, NaN, -0.05, 1.05],[.01, .01, NaN, .99, .99])
  UnitDelay3 : UnitDelay  SampleTime=-1  mask(TL_UnitDelay){data={'logdata',{'maxnumvals',4096,'plotchannels',[]},'output',{'type','Float32'},'state',{'type','Float32'},'date',735300.29227697919}}
      settings: CopyFcn=if exist('tl_reset_reviewflag','file')==2,tl_reset_reviewflag(gcbh);end  DeleteFcn=if exist('delete_tlblock','file')==2,delete_tlblock(gcbh);end  NameChangeFcn=if exist('rename_tlblock','file')==2,rename_tlblock(gcbh);end  OpenFcn=if exist('tl_open_blockdlg','file')==2,tl_open_blockdlg(gcbh);else,open_system(gcbh,'parameter');end
      mask Help: eval(['if exist(''tl_online_help'',''file'') == 2, tl_online_help(''Topic'',''TL_UnitDelay''),else, web([''jar:file:///'',matlabroot,''/help/toolbox/simulink/help.jar!/slref/' lower(get_param(gcbh,'Blocktype')) '.html''], ''-helpbrowser''),end'])
      mask Display: plot([-0.05, 1.05, NaN, -0.05, 1.05],[.01, .01, NaN, .99, .99])
  y : Outport
  wires:
  UnitDelay3/1 -> Product4/2
  Product2/1 -> Sum/1
  Product1/1 -> Sum/2
  UnitDelay2/1 -> Product2/1
  b2/1 -> Product2/2
  b1/1 -> Product1/2
  Product/1 -> Sum/3
  Product3/1 -> Sum/4
  a1/1 -> Product3/1
  b0/1 -> Product/2
  a2/1 -> Product4/1
  Product4/1 -> Sum/5
  UnitDelay/1 -> UnitDelay2/1, Product1/1
  u/1 -> UnitDelay/1, Product/1
  Sum/1 -> y/1, UnitDelay1/1
  UnitDelay1/1 -> Product3/2, UnitDelay3/1
